simulink model "simpleNN_S"  (R2021a)
settings: Solver=VariableStepAuto  StartTime=0.0  StopTime=10.0  RelTol=1e-3
libraries: neural x57
(part 2 of 2)

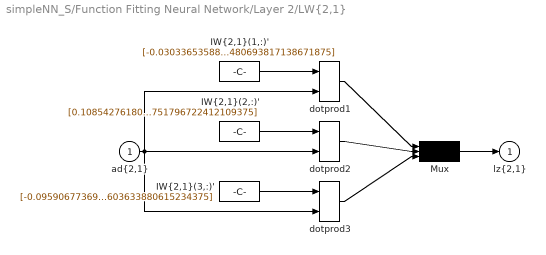
== system simpleNN_S/Function Fitting Neural Network/Layer 2/LW{2,1} ==
  "ad{2,1}" : Inport  PortDimensions=50
      mask Display: e = 0.06;c1 = [120 230 180]/255;c2 = ([120 230 180]+0)/(256+128);c3 = ([120 230 180]+128)/(256+128);patch([0 1 1 0],[0 0 1 1],c1);patch([0 1 1 1-e 1-e 0+e],[0 0 1 1-e 0+e 0+e],c2);patch([0 0 1 1-e 0+e 0+e],[0 1 1 1-e 1-e 0+e],c3);plot([0 1 1 0 0],[0 0 1 1 0]);
  "IW{2,1}(1,:)'" : Constant  Value=[-0.030336535880642667706297288532368838787078857421875;-0.056039902042742749388448686431729584001004695892333984375;0.360855970861353514411717924303957261145114898681640625;0.48866082200590577055976382325752638280391693115234375;0.0102889822954747855998647310116211883723735809326171875;-0.518626994384571826657293058815412223339080810546875;-0.279756323345283053338761192208039574325084686279296875;-0.047436559290216784301463803785736672580242156982421875;0.02676284339152039393194826288890908472239971160888671875;0.2213337557280153633509911514920531772077083587646484375;0.31827917195611210576799976479378528892993927001953125;-0.410557446594893293845274229170172475278377532958984375;0.073874783738018534595681785503984428942203521728515625;-0.34424502990603433882910167085356079041957855224609375;-0.1364242659677632474313213606365025043487548828125;0.0099534001820245389391406121148975216783583164215087890625;-1.0048713462678744434697364340536296367645263671875;-0.025318620904256849968305687070824205875396728515625;-0.026081332949036424573296955031764809973537921905517578125;-0.3755621090954559537777868172270245850086212158203125;-0.2315598502101373912243076347294845618307590484619140625;-0.071448570988844550821994516809354536235332489013671875;-0.03299428912674455538489581840622122399508953094482421875;0.051002342597788775935274685480180778540670871734619140625;0.16083618807276456319499402525252662599086761474609375;3.863221618278244395838783020735718309879302978515625;-0.183230446496017551627488728627213276922702789306640625;-0.05971082107608367828266437982165371067821979522705078125;-0.470116108479829986066533820121549069881439208984375;-0.288928403771399278099352159188129007816314697265625;0.51243600429878188862176102702505886554718017578125;-0.363964949244997504340659588706330396234989166259765625;0.01520098402391183156634468787160585634410381317138671875;0.14163417950678958145971364501747302711009979248046875;-0.2863123521782766633947403533966280519962310791015625;-0.36680673337229741104437152898753993213176727294921875;-0.338414359856806346016355746542103588581085205078125;-0.6421887552333400694948295495123602449893951416015625;-0.323235023197042448117599633405916392803192138671875;0.56474699907530634401808811162482015788555145263671875;-0.06626420211643306579230028319216216914355754852294921875;0.51407502993524423207105655819759704172611236572265625;0.6185939403928564228607456243480555713176727294921875;-0.42286235137863636968091896051191724836826324462890625;0.074281524999940895526151507510803639888763427734375;0.1221403125709873693782725467826821841299533843994140625;0.147598663703886134879184055535006336867809295654296875;-0.06680182712870187666798216241659247316420078277587890625;0.32501068401566446386397046808269806206226348876953125;-0.06344824600087987931384958528724382631480693817138671875]
      mask Display: e = 0.06;c1 = [120 150 230]/255;c2 = ([120 150 230]+0)/383;c3 = ([120 150 230]+128)/383;patch([0 1 1 0],[0 0 1 1],c1);patch([0 1 1 1-e 1-e 0+e],[0 0 1 1-e 0+e 0+e],c2);patch([0 0 1 1-e 0+e 0+e],[0 1 1 1-e 1-e 0+e],c3);plot([0 1 1 0 0],[0 0 1 1 0]);disp('weights');
  "IW{2,1}(2,:)'" : Constant  Value=[0.10854276180591186651280821706677670590579509735107421875;0.186956735295499443250122340032248757779598236083984375;1.012890560398770123384792896104045212268829345703125;0.002371342273922917576189917099327431060373783111572265625;0.1901929492633211982166585585218854248523712158203125;-0.457086643868093001064067948391311801970005035400390625;-0.059315487875708339249314349217456765472888946533203125;-0.019824694914804853740353252078421064652502536773681640625;-0.1028168533697009223715213011018931865692138671875;0.09571324114468271471167781783151440322399139404296875;0.186984668172556600662659320732927881181240081787109375;-0.062933060381354433143741289313766174018383026123046875;0.10900785219010121485094799709258950315415859222412109375;-0.08603605874076093729119207864641794003546237945556640625;-0.103500519898441556421175846480764448642730712890625;0.563829153547014794156666539493016898632049560546875;-0.27806342851226928392094350783736445009708404541015625;-0.0532568195149143164268679129236261360347270965576171875;-0.0178480682059896922364572446895181201398372650146484375;0.41656043482869542504687387918238528072834014892578125;0.17825836555823915130503110049176029860973358154296875;-0.090533129938662970648266536954906769096851348876953125;-0.02574033336175039765603145269778906367719173431396484375;0.189014642769497365204500738400383852422237396240234375;0.0396674487105695694477702772928751073777675628662109375;0.522256288445959171440335921943187713623046875;-0.313262616759330148052953290971345268189907073974609375;-0.01353461313063120119437598987133242189884185791015625;-0.0711682227822354740442989395887707360088825225830078125;0.00784270464390916799413133730922709219157695770263671875;0.129357071029643166948375210267840884625911712646484375;-0.340901511858545724908964302812819369137287139892578125;0.10230460898854527862500418677882407791912555694580078125;0.002434537711339772314556029186860541813075542449951171875;-0.1358292438027722537352559584178379736840724945068359375;0.06991593596316379721766764987478381954133510589599609375;-0.0018537452161906109449063251304323785006999969482421875;0.12736294522870583723062054559704847633838653564453125;0.022741079278333520274912871173000894486904144287109375;0.6483401983223051612270637633628211915493011474609375;0.058448701066409203264129246235825121402740478515625;-0.164363967979237524108526713462197221815586090087890625;-0.161756651636472514876885497869807295501232147216796875;0.0601907649117106313685354734843713231384754180908203125;0.329307148680577588262252675121999345719814300537109375;-0.139282267646020196938394519747816957533359527587890625;-0.0929612670950382968815262074713245965540409088134765625;-0.059509663364962668563595826753953588195145130157470703125;-0.025693017404758107524731514104132656939327716827392578125;-0.09445070859650817052255433736718259751796722412109375]
      mask Display: e = 0.06;c1 = [120 150 230]/255;c2 = ([120 150 230]+0)/383;c3 = ([120 150 230]+128)/383;patch([0 1 1 0],[0 0 1 1],c1);patch([0 1 1 1-e 1-e 0+e],[0 0 1 1-e 0+e 0+e],c2);patch([0 0 1 1-e 0+e 0+e],[0 1 1 1-e 1-e 0+e],c3);plot([0 1 1 0 0],[0 0 1 1 0]);disp('weights');
  "IW{2,1}(3,:)'" : Constant  Value=[-0.0959067736980395990631365066292346455156803131103515625;-0.078373749982505847011537980506545864045619964599609375;-0.83156361446387083713460697254049591720104217529296875;0.2433389369890023579134918918498442508280277252197265625;-0.25863650392163151092717043866286985576152801513671875;0.316614545929362611875745869838283397257328033447265625;0.0637758422492868959352563251741230487823486328125;-0.061671803620750635654967908294565859250724315643310546875;-0.0014760582393782695209694111326825805008411407470703125;0.2159216093839992633984792291812482289969921112060546875;-0.0750733094959772084830973426505806855857372283935546875;-0.1324632222461357144993598922155797481536865234375;0.0214018170493199821891039391630329191684722900390625;0.1702981465227537405393576364076579920947551727294921875;-0.0073156767559848685789081201846784097142517566680908203125;0.210160646180505727986798092388198710978031158447265625;-0.2478300397176197156223764750393456779420375823974609375;-0.03376324302192824922119740449488745070993900299072265625;-0.1783296996789574262454181052817148156464099884033203125;-0.1947188191654928013374359352383180521428585052490234375;0.0114513694512690944460331365917227230966091156005859375;0.281379737417346564853914969717152416706085205078125;-0.084373211075543519399388969759456813335418701171875;-0.0388061044256925169460004099164507351815700531005859375;0.59075769811051603852547486894764006137847900390625;-2.95923255671147433787382396985776722431182861328125;0.2322402050726515287948359400616027414798736572265625;0.0774829836223590862065435658223577775061130523681640625;0.10218186305466696317534314175645704381167888641357421875;0.28907326809289257685264828978688456118106842041015625;-0.1604770330109669129736715831313631497323513031005859375;0.168323808455431100927768284236663021147251129150390625;0.07222581823278113877240258489109692163765430450439453125;0.03586904109784892769052788707995205186307430267333984375;-0.26234613341312151835182930881273932754993438720703125;0.185212312661103606359347395482473075389862060546875;0.1163228871188017043980522657875553704798221588134765625;-0.083177508486260876008344666843186132609844207763671875;0.2603532064215874353152457842952571809291839599609375;-0.3344594874920965299480712928925640881061553955078125;0.02780100096433264778017502294460427947342395782470703125;0.38521060625183178860453381275874562561511993408203125;0.266100434701464216846744648137246258556842803955078125;0.41189370845812700583365995044005103409290313720703125;-0.371993819874496145505560207311646081507205963134765625;-0.08150451239148805149259402469397173263132572174072265625;0.05550130638846988151424710622450220398604869842529296875;0.00379761730184053312997516371751771657727658748626708984375;0.082078247944954052517374520903103984892368316650390625;0.413842501274602037053540470878942869603633880615234375]
      mask Display: e = 0.06;c1 = [120 150 230]/255;c2 = ([120 150 230]+0)/383;c3 = ([120 150 230]+128)/383;patch([0 1 1 0],[0 0 1 1],c1);patch([0 1 1 1-e 1-e 0+e],[0 0 1 1-e 0+e 0+e],c2);patch([0 0 1 1-e 0+e 0+e],[0 1 1 1-e 1-e 0+e],c3);plot([0 1 1 0 0],[0 0 1 1 0]);disp('weights');
  Mux : Mux  Inputs=3
      mask Display: e = 0.06;c1 = [120 150 230]/255;c2 = ([120 150 230]+0)/383;c3 = ([120 150 230]+128)/383;patch([0 1 1 0],[0 0 1 1],c1);patch([0 1 1 1-e 1-e 0+e],[0 0 1 1-e 0+e 0+e],c2);patch([0 0 1 1-e 0+e 0+e],[0 1 1 1-e 1-e 0+e],c3);plot([0 1 1 0 0],[0 0 1 1 0]);disp('Mux');
  dotprod1 : neural/Weight Functions/dotprod
  dotprod2 : neural/Weight Functions/dotprod
  dotprod3 : neural/Weight Functions/dotprod
  "lz{2,1}" : Outport
      mask Display: e = 0.06;c1 = [120 230 180]/255;c2 = ([120 230 180]+0)/(256+128);c3 = ([120 230 180]+128)/(256+128);patch([0 1 1 0],[0 0 1 1],c1);patch([0 1 1 1-e 1-e 0+e],[0 0 1 1-e 0+e 0+e],c2);patch([0 0 1 1-e 0+e 0+e],[0 1 1 1-e 1-e 0+e],c3);plot([0 1 1 0 0],[0 0 1 1 0]);
  wires:
  "IW{2,1}(1,:)'"/1 -> dotprod1/1
  "ad{2,1}"/1 -> dotprod1/2, dotprod2/2, dotprod3/2
  dotprod1/1 -> Mux/1
  "IW{2,1}(2,:)'"/1 -> dotprod2/1
  dotprod2/1 -> Mux/2
  "IW{2,1}(3,:)'"/1 -> dotprod3/1
  dotprod3/1 -> Mux/3
  Mux/1 -> "lz{2,1}"/1
